simulink model "raw2jointDemo"  (R2016b)
settings: Solver=ode5  StartTime=0.0  StopTime=20  FixedStep=0.001  RelTol=1e-3  EnableMultiTasking=on
libraries: dcpctrl x4
settings Model: SimulationMode=external  Creator=julianleland  LastModifiedBy=julianleland
settings OptimizationCC: LifeSpan=inf
settings DebuggingCC: SFUnexpectedBacktrackingDiag=warning  SFNoUnconditionalDefaultTransitionDiag=warning  SFExecutionAtInitializationDiag=none
settings HardwareCC: ProdBitPerLong=64  ProdHWDeviceType=Intel->x86-64 (Mac OS X)  TargetBitPerLong=64  TargetBitPerPointer=64  TargetIntDivRoundTo=Zero  TargetEndianess=LittleEndian  TargetWordSize=64  TargetHWDeviceType=Intel->x86-64
settings RTWCC: SystemTargetFile=sldrt.tlc  TemplateMakefile=sldrt.tmf  Description=Simulink Desktop Real-Time  RTWCompilerOptimization=on
settings CodeAppCC: MaxIdLength=95
settings SimulinkDesktopRealTimeCC: TargetPreCompLibLocation=/Applications/MATLAB_R2016b.app/toolbox/sldrt/lib/maci64  TargetLangStandard=C89/C90 (ANSI)  SupportVariableSizeSignals=off
settings ConfigComp: CovMetricSettings=dw  CovHtmlReporting=on  CovSaveCumulativeToWorkspaceVar=on  CovSaveSingleToWorkspaceVar=on  CovExternalEMLEnable=off

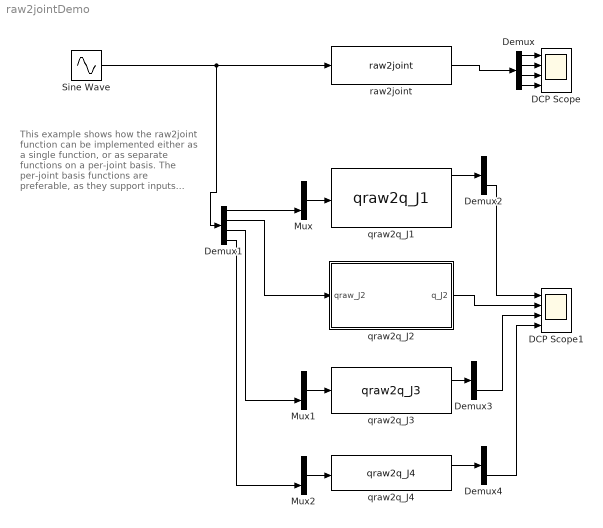
== system raw2jointDemo ==
  note: This example shows how the raw2joint function can be implemented either as a single function, or as separate functions on a per-joint basis. The per-joint basis functions are preferable, as they support inputs from absolute & relative encoders
  DCP Scope : Scope  NumInputPorts=4
  DCP Scope1 : Scope  NumInputPorts=4
  Demux : Demux
  Demux1 : Demux
  Demux2 : Demux  Outputs=2
  Demux3 : Demux  Outputs=2
  Demux4 : Demux  Outputs=2
  Mux : Mux  Inputs=2
  Mux1 : Mux  Inputs=2
  Mux2 : Mux  Inputs=2
  Sine Wave : Sin  Amplitude=[5 6 4 7]  SampleTime=0
  qraw2q_J1 : dcpctrl/qraw2q_J1
  qraw2q_J2 : Subsystem
  qraw2q_J3 : dcpctrl/qraw2q_J3
  qraw2q_J4 : dcpctrl/qraw2q_J4
  raw2joint : dcpctrl/raw2joint
  wires:
  Sine Wave/1 -> Demux1/1, raw2joint/1
  Demux/1 -> DCP Scope/1
  Demux/2 -> DCP Scope/2
  Demux/3 -> DCP Scope/3
  Demux/4 -> DCP Scope/4
  raw2joint/1 -> Demux/1
  Mux/1 -> qraw2q_J1/1
  Demux1/1 -> Mux/2
  Mux1/1 -> qraw2q_J3/1
  Mux2/1 -> qraw2q_J4/1
  Demux1/4 -> Mux2/2
  Demux1/3 -> Mux1/2
  Demux1/2 -> qraw2q_J2/1(qraw_J2)
  Demux2/2 -> DCP Scope1/1
  Demux4/2 -> DCP Scope1/4
  qraw2q_J1/1 -> Demux2/1
  qraw2q_J4/1 -> Demux4/1
  qraw2q_J3/1 -> Demux3/1
  qraw2q_J2/1(q_J2) -> DCP Scope1/2
  Demux3/2 -> DCP Scope1/3

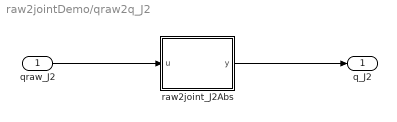
== system raw2jointDemo/qraw2q_J2 ==
  qraw_J2 : Inport
  raw2joint_J2Abs : MATLAB Function  TreatAsAtomicUnit=on
  q_J2 : Outport
  wires:
  raw2joint_J2Abs/1(y) -> q_J2/1
  qraw_J2/1 -> raw2joint_J2Abs/1(u)

== matlab function raw2jointDemo/qraw2q_J2/raw2joint_J2Abs ==
  data: u input; y output; robot parameter
function y = fcn(u,robot)

%#codegen

y_temp = raw2jointJ2Abs_at40gw(robot,u');
y = y_temp';
